simulink model "MVC4"  (R2019b)
settings: Solver=VariableStepAuto  StartTime=0.0  StopTime=SimulationTime  RelTol=1e-3
values from neighbouring files (symbols this model uses):
  disturbanceStrength = 0.001    [Obliczenia.m]
  RegulatedValue = 5    [Obliczenia.m]
  SampleTime = 1    [Obliczenia.m]
libraries: simulink x5
settings Model: Creator=pleka  LastModifiedBy=pleka

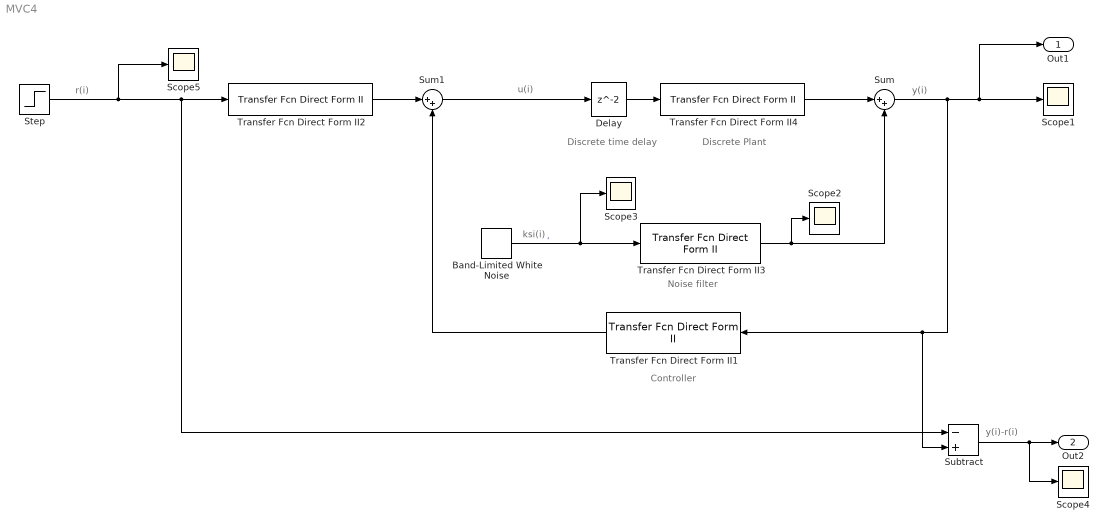
== system MVC4 ==
  note: Discrete Plant
  note: u(i)
  note: Discrete time delay
  note: Noise filter
  note: Controller
  note: r(i)
  note: y(i)-r(i)
  note: y(i)
  note: ksi(i)
  Band-Limited White Noise : simulink/Sources/Band-Limited White Noise  Cov=[disturbanceStrength]  Ts=SampleTime  seed=[23341]
  Delay : Delay
  Scope{1..5} (5 alike) : Scope
  Step : Step  After=RegulatedValue  SampleTime=SampleTime
  Subtract : Sum  Inputs=-+
  Sum : Sum  Inputs=|++
  Sum1 : Sum  Inputs=|++
  Transfer Fcn Direct Form II1 : simulink/Additional Math & Discrete/Additional Discrete/Transfer Fcn Direct Form II  NumCoefVec=[-81 0]  DenCoefVec=[0.9]  vinit=0.0  DoSatur=off
      settings: SourceProductName=Simulink  SourceProductBaseCode=SL
  Transfer Fcn Direct Form II2 : simulink/Additional Math & Discrete/Additional Discrete/Transfer Fcn Direct Form II  NumCoefVec=[100 0]  DenCoefVec=[0.9]  vinit=0.0  DoSatur=off
      settings: SourceProductName=Simulink  SourceProductBaseCode=SL
  Transfer Fcn Direct Form II3 : simulink/Additional Math & Discrete/Additional Discrete/Transfer Fcn Direct Form II  NumCoefVec=[1 0]  DenCoefVec=[-0.9]  vinit=0.0  DoSatur=off
      settings: SourceProductName=Simulink  SourceProductBaseCode=SL
  Transfer Fcn Direct Form II4 : simulink/Additional Math & Discrete/Additional Discrete/Transfer Fcn Direct Form II  NumCoefVec=[0.01 0]  DenCoefVec=[-0.9]  vinit=0.0  DoSatur=off
      settings: SourceProductName=Simulink  SourceProductBaseCode=SL
  Out1 : Outport
  Out2 : Outport  Port=2
  wires:
  Step/1 -> Subtract/1, Transfer Fcn Direct Form II2/1, Scope5/1
  Sum1/1 -> Delay/1
  Transfer Fcn Direct Form II3/1 -> Scope2/1, Sum/2
  Transfer Fcn Direct Form II2/1 -> Sum1/1
  Sum/1 -> Subtract/2, Transfer Fcn Direct Form II1/1, Out1/1, Scope1/1
  Band-Limited White Noise/1 -> Transfer Fcn Direct Form II3/1, Scope3/1  ","
  Transfer Fcn Direct Form II1/1 -> Sum1/2
  Subtract/1 -> Scope4/1, Out2/1
  Transfer Fcn Direct Form II4/1 -> Sum/1
  Delay/1 -> Transfer Fcn Direct Form II4/1
